simulink model "integrationTest1"  (R2018a)
settings: Solver=VariableStepAuto  StartTime=0.0  StopTime=10.0  RelTol=1e-3
settings Model: Creator=ppatil  LastModifiedBy=ppatil

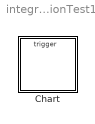
== system integrationTest1 ==
  Chart : Stateflow chart  TreatAsAtomicUnit=on

== stateflow chart integrationTest1/Chart ==
  state A [parallel]
    settings: executionOrder=1
    state A
      state A [parallel]
        en:
        countVal = count(loc1>0);
        inVal = in(A.A.A);
        tickVal = 1;
        on after(1, tick):
        tickVal = tickVal+1;
        on after(loc1+loc2, tick):
        tickVal = tickVal+1;
        on after(1, E1):
        tickVal = tickVal+1;
        on after(loc1+loc2, E1):
        tickVal = tickVal+1;
        settings: executionOrder=1
      state B [parallel]
        settings: executionOrder=2
    state B
      state A
      state B
      state C
      state D
      (default) -> A.B.A
      A.B.A -> (junction 39) [order 1]
      (junction 39) -> A.B.B [order 1]
      (junction 39) -> (junction 41) [order 2]
      A.B.B -> A.B.A
      A.B.A -> D [order 2]
      D -> A.B.A
      (junction 41) -> A.B.C [order 1]
    state C
    (default) -> A.A
    A.A -> A.B [order 1] : at(3, sec)[tickVal==1]
    A.B -> A.A
    A.A -> A.B.B [order 2] : at(3,sec){tickVfal=20}
    (junction 41) -> A.C [order 2]
    A.C -> A.B
  (default) -> A
  data: loc1 local =1; loc2 local =1; countVal local; inVal local; tickVal local
  events: E1 input RISING_EDGE_EVENT
